simulink model "Compare_lin_nonlin"  (R2021b)
settings: Solver=VariableStepAuto  StartTime=0.0  StopTime=10  RelTol=1e-3
values from neighbouring files (symbols this model uses):
  eq_perturbed = stateToSimulinkOrder([0, 0, -perturbation, 0])    [Linearization_comparison.m]
  g = 9.81    [init.m]
  L = 2    [init.m]
  M = 5    [init.m]
  m = 1    [init.m]
  theta0 = pi    (= 3.14159265359)    [Linearization_comparison.m]
  theta_perturbed = theta0 - perturbation    (= 2.99159265359)    [Linearization_comparison.m]    (also in Synthesis.m)
undefined symbols (not defined in the file or in its folder): A, B, C, D
settings Model: Creator=fabri  LastModifiedBy=brizio
settings DebuggingCC: UnconnectedInputMsg=none  UnconnectedOutputMsg=none  UnconnectedLineMsg=none
settings ModelReferenceCC: EnableRefExpFcnMdlSchedulingChecks=off
settings RTWCC: DLArmComputeVersion=20.02.1

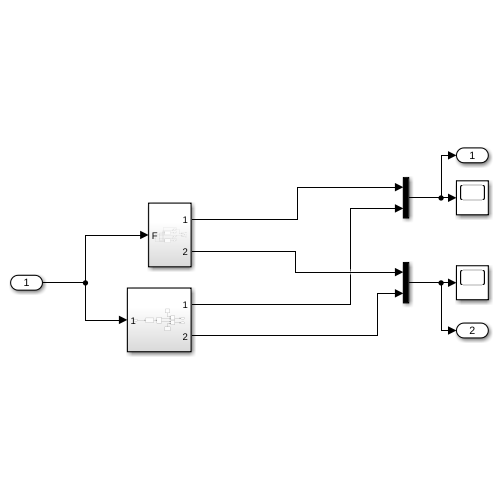
[thumbnail: Simulink's stored preview of the top-level diagram]
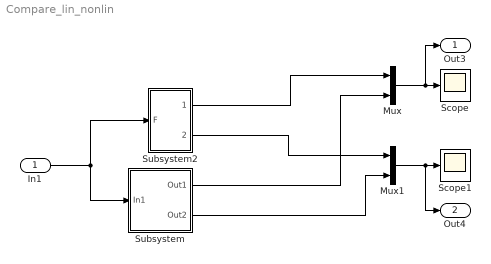
== system Compare_lin_nonlin ==
  In1 : Inport
  Mux : Mux  Inputs=2
  Mux1 : Mux  Inputs=2
  Scope : Scope
  Scope1 : Scope
  Subsystem : Subsystem
  Subsystem2 : Subsystem
  Out3 : Outport
  Out4 : Outport  Port=2
  wires:
  In1/1 -> Subsystem/1(In1), Subsystem2/1(F)
  Mux1/1 -> Out4/1, Scope1/1
  Mux/1 -> Out3/1, Scope/1
  Subsystem2/1(Out1) -> Mux/1
  Subsystem/1(Out1) -> Mux/2
  Subsystem2/2(Out2) -> Mux1/1
  Subsystem/2(Out2) -> Mux1/2

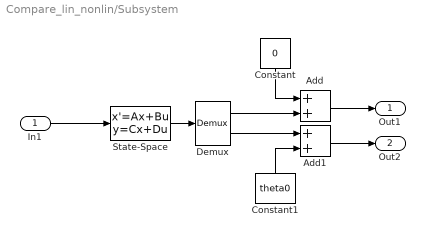
== system Compare_lin_nonlin/Subsystem ==
  In1 : Inport
  Add : Sum
  Add1 : Sum
  Constant : Constant  Value=0
  Constant1 : Constant  Value=theta0
  Demux : Demux  Outputs=2
      settings: DisplayOption=none
  State-Space : StateSpace  A=A  B=B  C=C  D=D  InitialCondition=eq_perturbed
  Out1 : Outport
  Out2 : Outport  Port=2
  wires:
  In1/1 -> State-Space/1
  State-Space/1 -> Demux/1
  Demux/2 -> Add1/1
  Demux/1 -> Add/2
  Add1/1 -> Out2/1
  Add/1 -> Out1/1
  Constant/1 -> Add/1
  Constant1/1 -> Add1/2

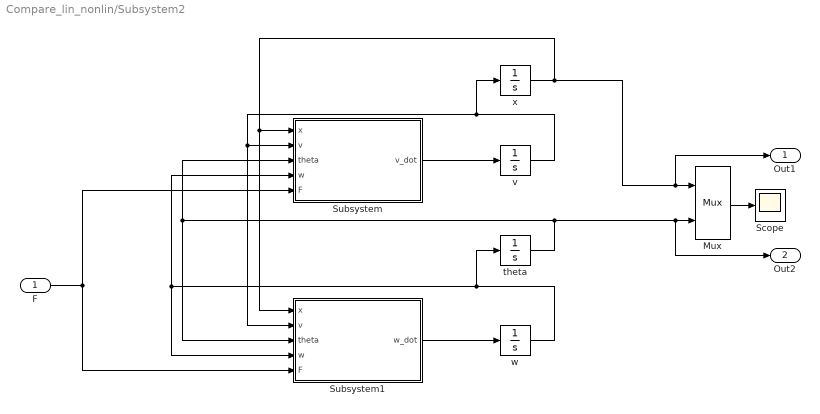
== system Compare_lin_nonlin/Subsystem2 ==
  F : Inport
  Mux : Mux  Inputs=2
      settings: DisplayOption=signals
  Scope : Scope
  Subsystem : Subsystem
  Subsystem1 : Subsystem
  theta : Integrator  InitialCondition=theta_perturbed
  v : Integrator
  w : Integrator
  x : Integrator
  Out1 : Outport
  Out2 : Outport  Port=2
  wires:
  Subsystem1/1(w_dot) -> w/1
  F/1 -> Subsystem/5(F), Subsystem1/5(F)
  x/1 -> Out1/1, Mux/1, Subsystem1/1(x), Subsystem/1(x)
  v/1 -> Subsystem/2(v), Subsystem1/2(v), x/1
  w/1 -> Subsystem1/4(w), Subsystem/4(w), theta/1
  theta/1 -> Subsystem/3(theta), Subsystem1/3(theta), Out2/1, Mux/2
  Mux/1 -> Scope/1
  Subsystem/1(v_dot) -> v/1

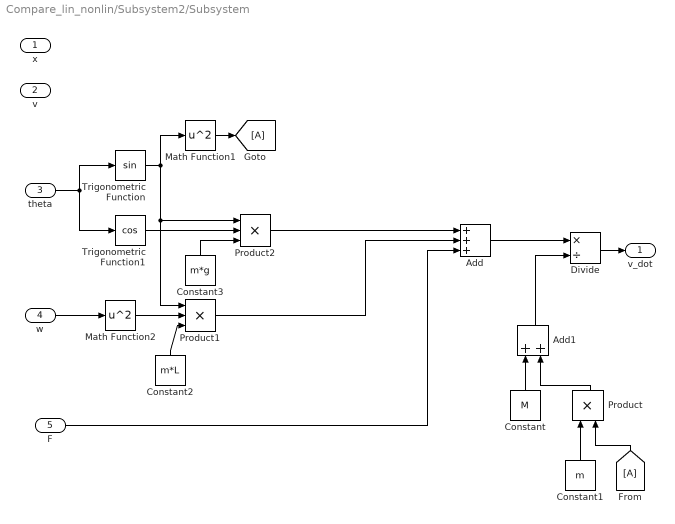
== system Compare_lin_nonlin/Subsystem2/Subsystem ==
  x : Inport
  v : Inport  Port=2
  theta : Inport  Port=3
  w : Inport  Port=4
  F : Inport  Port=5
  Add : Sum  Inputs=+++
  Add1 : Sum
  Constant : Constant  Value=M
  Constant1 : Constant  Value=m
  Constant2 : Constant  Value=m*L
  Constant3 : Constant  Value=m*g
  Divide : Product  Inputs=*/
  Math Function1 : Math  Operator=square  SaturateOnIntegerOverflow=on
  Math Function2 : Math  Operator=square  SaturateOnIntegerOverflow=on
  Product : Product
  Product1 : Product  Inputs=3
  Product2 : Product  Inputs=3
  Trigonometric Function : Trigonometry
  Trigonometric Function1 : Trigonometry  Operator=cos
  v_dot : Outport
  wires:
  Divide/1 -> v_dot/1
  Add1/1 -> Divide/2
  Constant/1 -> Add1/1
  Product/1 -> Add1/2
  theta/1 -> Trigonometric Function1/1, Trigonometric Function/1
  Trigonometric Function/1 -> Product1/1, Product2/1, Math Function1/1
  w/1 -> Math Function2/1
  Math Function1/1 -> [A]
  [A] -> Product/2
  Constant1/1 -> Product/1
  Math Function2/1 -> Product1/2
  Constant2/1 -> Product1/3
  Add/1 -> Divide/1
  Trigonometric Function1/1 -> Product2/2
  Constant3/1 -> Product2/3
  Product1/1 -> Add/2
  Product2/1 -> Add/1
  F/1 -> Add/3

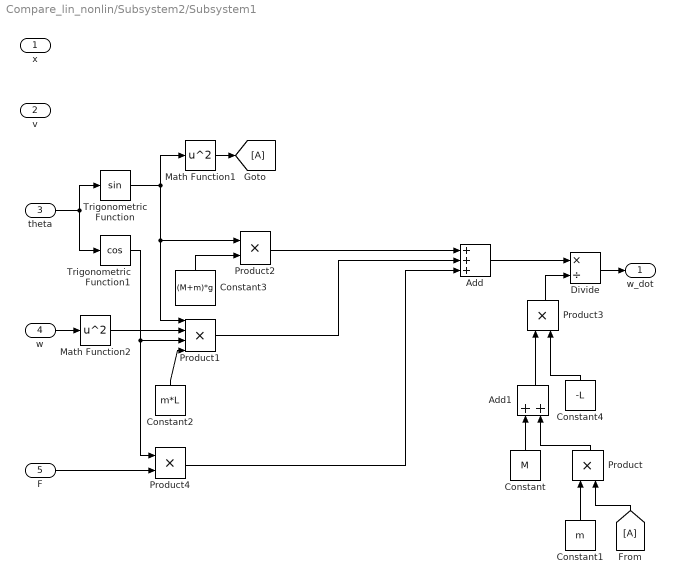
== system Compare_lin_nonlin/Subsystem2/Subsystem1 ==
  x : Inport
  v : Inport  Port=2
  theta : Inport  Port=3
  w : Inport  Port=4
  F : Inport  Port=5
  Add : Sum  Inputs=+++
  Add1 : Sum
  Constant : Constant  Value=M
  Constant1 : Constant  Value=m
  Constant2 : Constant  Value=m*L
  Constant3 : Constant  Value=(M+m)*g
  Constant4 : Constant  Value=-L
  Divide : Product  Inputs=*/
  Math Function1 : Math  Operator=square  SaturateOnIntegerOverflow=on
  Math Function2 : Math  Operator=square  SaturateOnIntegerOverflow=on
  Product{,2..4} (4 alike) : Product
  Product1 : Product  Inputs=4
  Trigonometric Function : Trigonometry
  Trigonometric Function1 : Trigonometry  Operator=cos
  w_dot : Outport
  wires:
  Divide/1 -> w_dot/1
  Constant/1 -> Add1/1
  Product/1 -> Add1/2
  theta/1 -> Trigonometric Function1/1, Trigonometric Function/1
  Trigonometric Function/1 -> Product1/1, Product2/1, Math Function1/1
  w/1 -> Math Function2/1
  Math Function1/1 -> [A]
  [A] -> Product/2
  Constant1/1 -> Product/1
  Math Function2/1 -> Product1/2
  Add/1 -> Divide/1
  Trigonometric Function1/1 -> Product1/3, Product4/1
  Constant3/1 -> Product2/2
  Product1/1 -> Add/2
  Product2/1 -> Add/1
  Add1/1 -> Product3/1
  Product3/1 -> Divide/2
  Constant4/1 -> Product3/2
  F/1 -> Product4/2
  Product4/1 -> Add/3
  Constant2/1 -> Product1/4
